simulink subsystem "PieroModel"  (R2023b)
settings: Solver=VariableStepAuto  StartTime=0.0  StopTime=10.0  RelTol=1e-3
settings Model: Creator=Felix  LastModifiedBy=Daniel

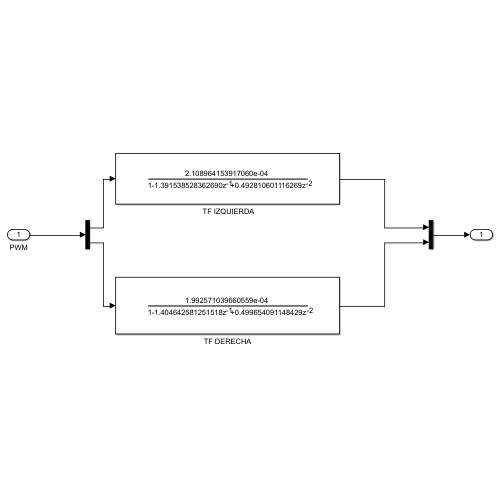
[thumbnail: Simulink's stored preview of the top-level diagram]
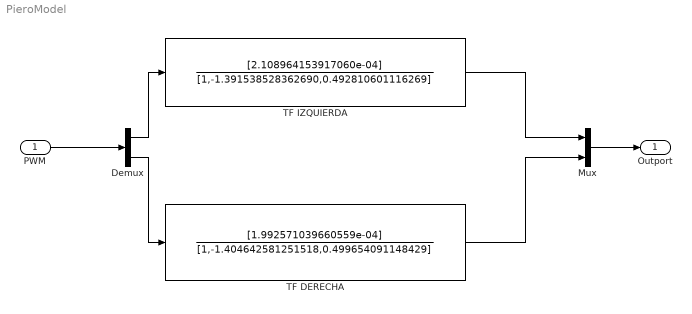
== system PieroModel ==
  PWM : Inport
  " TF IZQUIERDA" : DiscreteFilter  Numerator=[2.108964153917060e-04]  Denominator=[1,-1.391538528362690,0.492810601116269]
  Demux : Demux  Outputs=2
  Mux : Mux  Inputs=2
  TF DERECHA : DiscreteFilter  Numerator=[1.992571039660559e-04]  Denominator=[1,-1.404642581251518,0.499654091148429]
  Outport : Outport
  wires:
  PWM/1 -> Demux/1
  Mux/1 -> Outport/1
  Demux/1 -> " TF IZQUIERDA"/1
  Demux/2 -> TF DERECHA/1
  " TF IZQUIERDA"/1 -> Mux/1
  TF DERECHA/1 -> Mux/2
